simulink model "twopots"  (R2021b)
settings: Solver=FixedStepAuto  StartTime=0.0  StopTime=Inf  RelTol=1e-3
libraries: arduinolib x2
settings Model: ExtModeTrigDuration=2  Creator=cirie  LastModifiedBy=cirie
settings OptimizationCC: EnhancedBackFolding=on  PassReuseOutputArgsAs=Individual arguments  ZeroExternalMemoryAtStartup=off  ZeroInternalMemoryAtStartup=off  MaxStackSize=64  OptimizeBlockOrder=speed  DifferentSizesBufferReuse=on  OptimizationCustomize=off  EfficientTunableParamExpr=on
settings DebuggingCC: ParameterTunabilityLossMsg=error
settings HardwareCC: ProdBitPerPointer=32  ProdBitPerSizeT=32  ProdBitPerPtrDiffT=32  ProdLargestAtomicInteger=Long  ProdLargestAtomicFloat=Double  ProdWordSize=32  ProdHWDeviceType=ARM Compatible->ARM Cortex
settings SFSimCC: MATLABDynamicMemAlloc=off
settings RTWCC: Description=Embedded Coder  SystemTargetFile=ert.tlc  HardwareBoard=Arduino MKR WiFi 1010  TemplateMakefile=ert_default_tmf  Toolchain=Arduino ARM
settings CodeAppCC: ForceParamTrailComments=on  IgnoreCustomStorageClasses=off  OperatorAnnotations=on  SimulinkDataObjDesc=on  SFDataObjDesc=on  InsertBlockDesc=on
settings ERTTargetCC: SupportContinuousTime=on  SupportVariableSizeSignals=on  ExtModeTransport=3  ExtModeStaticAlloc=on  ExtModeStaticAllocSize=8192  ExtModeMexFile=ext_xcp  ExtModeIntrfLevel=Level2 - Open

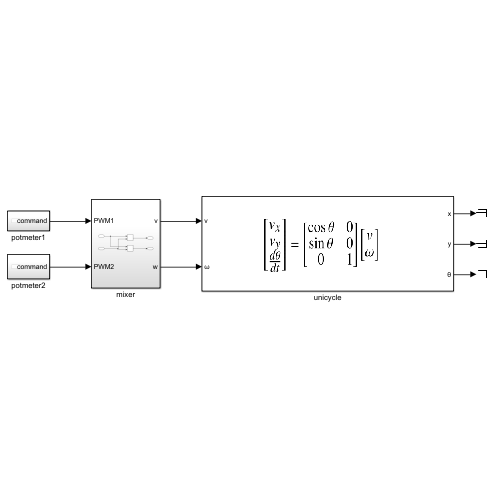
[thumbnail: Simulink's stored preview of the top-level diagram]
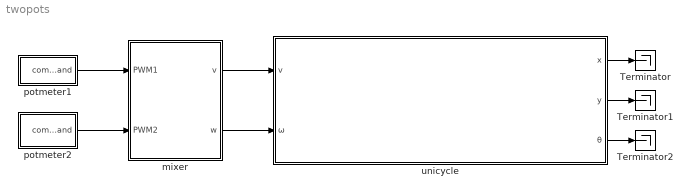
== system twopots ==
  Terminator : Terminator
  Terminator1 : Terminator
  Terminator2 : Terminator
  mixer : Subsystem
  potmeter1 : Subsystem
  potmeter2 : Subsystem
  unicycle : Subsystem
      mask Display: image('$imagefile'); % Use "Edit Image" on toolstrip to change.
  wires:
  potmeter1/1(command) -> mixer/1(PWM1)
  potmeter2/1(command) -> mixer/2(PWM2)
  mixer/1(v) -> unicycle/1(v)
  mixer/2(w) -> unicycle/2(ω)
  unicycle/1(x) -> Terminator/1
  unicycle/2(y) -> Terminator1/1
  unicycle/3(θ) -> Terminator2/1

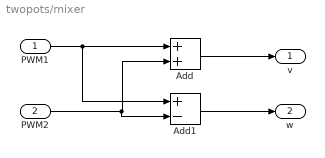
== system twopots/mixer ==
  PWM1 : Inport
  PWM2 : Inport  Port=2
  Add : Sum
  Add1 : Sum  Inputs=+-
  v : Outport
  w : Outport  Port=2
  wires:
  PWM1/1 -> Add1/1, Add/1
  PWM2/1 -> Add1/2, Add/2
  Add/1 -> v/1
  Add1/1 -> w/1

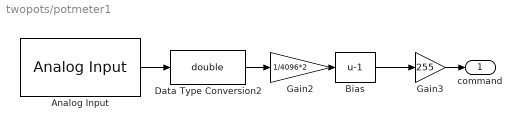
== system twopots/potmeter1 ==
  Analog Input : arduinolib/Analog Input  pinNumber=5  ReadResultsOnly=off  ConversionTriggerSource=Software  ExternalTriggerType=uint32( 0 )  OutputDataType=uint16  EnableConversionCompleteNotify=off  EnableOuputStatus=off  SampleTime=-1  blockPlatform=arduino
  Bias : Bias  Bias=-1
  Data Type Conversion2 : DataTypeConversion  OutDataTypeStr=double
  Gain2 : Gain  Gain=1/4096*2
  Gain3 : Gain  Gain=255
  command : Outport
  wires:
  Bias/1 -> Gain3/1
  Data Type Conversion2/1 -> Gain2/1
  Analog Input/1 -> Data Type Conversion2/1
  Gain2/1 -> Bias/1
  Gain3/1 -> command/1

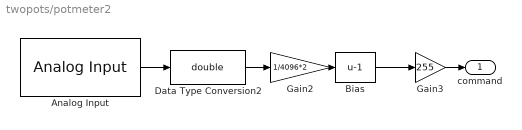
== system twopots/potmeter2 ==
  Analog Input : arduinolib/Analog Input  pinNumber=4  ReadResultsOnly=off  ConversionTriggerSource=Software  ExternalTriggerType=uint32( 0 )  OutputDataType=uint16  EnableConversionCompleteNotify=off  EnableOuputStatus=off  SampleTime=-1  blockPlatform=arduino
  Bias : Bias  Bias=-1
  Data Type Conversion2 : DataTypeConversion  OutDataTypeStr=double
  Gain2 : Gain  Gain=1/4096*2
  Gain3 : Gain  Gain=255
  command : Outport
  wires:
  Gain3/1 -> command/1
  Gain2/1 -> Bias/1
  Analog Input/1 -> Data Type Conversion2/1
  Data Type Conversion2/1 -> Gain2/1
  Bias/1 -> Gain3/1

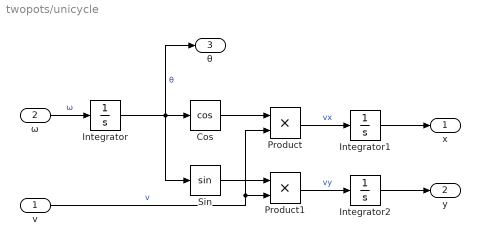
== system twopots/unicycle ==
  v : Inport
  ω : Inport  Port=2
  Cos : Trigonometry  Operator=cos
  Integrator : Integrator
  Integrator1 : Integrator
  Integrator2 : Integrator
  Product : Product
  Product1 : Product
  Sin : Trigonometry
  x : Outport
  y : Outport  Port=2
  θ : Outport  Port=3
  wires:
  ω/1 -> Integrator/1  "ω"
  Sin/1 -> Product1/1
  Integrator1/1 -> x/1
  Cos/1 -> Product/1
  Integrator/1 -> θ/1, Sin/1, Cos/1  "θ"
  Product/1 -> Integrator1/1  "vx"
  Product1/1 -> Integrator2/1  "vy"
  v/1 -> Product/2, Product1/2  "v"
  Integrator2/1 -> y/1
